simulink model "RLInvertedPendulumCtrl"  (R2017a)
settings: Solver=ode5  StartTime=0.0  StopTime=60  FixedStep=0.01  RelTol=1e-3
PreLoadFcn:
  | InvertedPendulumCtrlInit
values from neighbouring files (symbols this model uses):
  eta = 1.05    [InvertedPendulumSimCtrlInit.m]
  g = 9.81    [PendulumParameters.m]
  J = 0.0087878516209625    (= 0.00878785162096)    [PendulumParameters.m]
  K = lqr(A, B, Q, R)    [InvertedPendulumSimCtrlInit.m]
  kcw = 3    [InvertedPendulumSimCtrlInit.m]
  kem = 7    [InvertedPendulumSimCtrlInit.m]
  ksu = 1.3    [InvertedPendulumSimCtrlInit.m]
  kvw = 3    [InvertedPendulumSimCtrlInit.m]
  l = 0.2545253256150507    (= 0.254525325615)    [PendulumParameters.m]    (also in PlotPendulum.m = 1.8)
  mp = 0.096739999999999999    (= 0.09674)    [PendulumParameters.m]
  OffsetCart = 0    [PendulumParameters.m]
  OffsetPend = pi    (= 3.14159265359)    [PendulumParameters.m]
  ResCartEnc = 0.235 / 4096    (= 5.7373046875e-05)    [PendulumParameters.m]
  ResPendEnc = 2 * pi / 4096    (= 0.00153398078789)    [PendulumParameters.m]
  Td = 0.0    (= 0)    [InvertedPendulumSimCtrlInit.m]
  Ts = 0.01    [PendulumParameters.m]
  vmax = 5    [InvertedPendulumSimCtrlInit.m]
  x0 = [0; 0; pi + 0.01; 0]    [InvertedPendulumSimCtrlInit.m]
  xmax = 0.4    [InvertedPendulumSimCtrlInit.m]
undefined symbols (not defined in the file or in its folder): bias, bias0, bias2, bias4, M, sgn, weight0, weight2, weight4
undefined symbols (not defined in the file): angleSZ, Fs, RTDAC4PCIBaseAddress
libraries: simulink x1
settings Model: SimulationMode=external  ExtModeTrigDuration=12000  ExtModeTrigLevel=0.400000  Creator=jims  LastModifiedBy=Pendulum
settings DataIOCC: SaveFormat=Array  SaveOutput=off  SignalLogging=off  DSMLogging=off  SaveTime=off  SignalLoggingName=sigsOut
settings OptimizationCC: DefaultParameterBehavior=Inlined  InlineInvariantSignals=on  EfficientFloat2IntCast=on  SimCompilerOptimization=on
settings DebuggingCC: SaveWithParameterizedLinksMsg=none  IntegerOverflowMsg=none  UniqueDataStoreMsg=error  AssertControl=DisableAll  StrictBusMsg=ErrorOnBusTreatedAsVector  SFUnexpectedBacktrackingDiag=warning  SFNoUnconditionalDefaultTransitionDiag=warning  SFExecutionAtInitializationDiag=none  IntegerSaturationMsg=none
settings ModelReferenceCC: PropagateSignalLabelsOutOfModel=off
settings SFSimCC: SimParseCustomCode=off
settings RTWCC: SystemTargetFile=sldrt.tlc  TemplateMakefile=sldrt.tmf  Description=Simulink Desktop Real-Time  RTWCompilerOptimization=on
settings CodeAppCC: MaxIdLength=95
settings SimulinkDesktopRealTimeCC: TargetPreCompLibLocation=C:\Program Files\MATLAB\R2017a\toolbox\sldrt\lib\win64  TargetLangStandard=C89/C90 (ANSI)  SupportVariableSizeSignals=off
settings ConfigComp: CovMetricSettings=dw  CovHtmlReporting=on  CovSaveCumulativeToWorkspaceVar=on  CovSaveSingleToWorkspaceVar=on  CovExternalEMLEnable=off  CovSFcnEnable=off

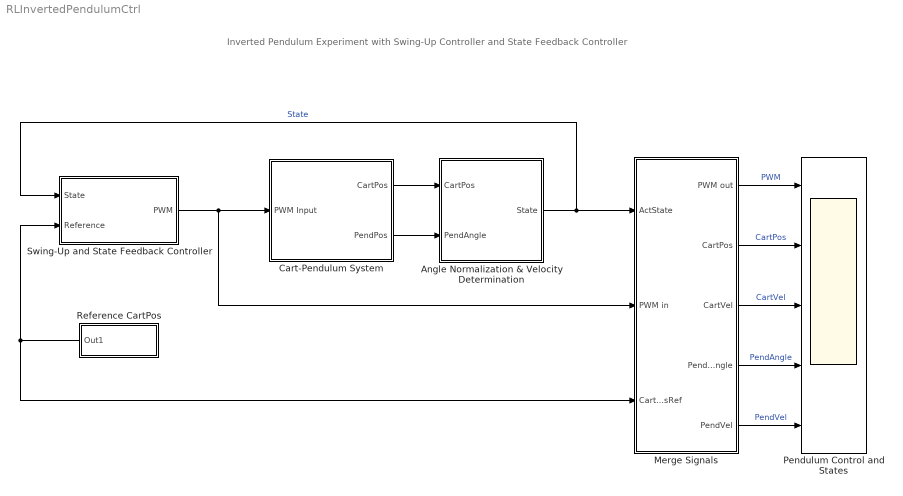
== system RLInvertedPendulumCtrl ==
  note: Inverted Pendulum Experiment with
      | Swing-Up Controller and State Feedback Controller
  Angle Normalization & Velocity Determination : Subsystem
  Cart-Pendulum System : Subsystem  mask(Cart-Pendulum System){BaseAddress=RTDAC4PCIBaseAddress(-1,-1)}
      mask prompts: BaseAddress "Base Address:"
      mask help: Interface to Cart-Pendulum System
      mask Display:
      | plot( [0.725 0.725], [1.15 0.375]); % pendulum arm
      | plot(0.725+0.05*sin([0:0.5:7]), 0.325+0.05*cos([0:0.5:7])); % pendulum load mass
      | plot([-0.2], [-0.2]);
      | plot([1.9], [1.7]);
      | plot([0.1 1.4], [1.09 1.09]); % upper rail
      | plot([0.1 1.4], [1.07 1.07]); % upper rail
      | plot([0.65 0.8], [1.1 1.1]); % cart bottom
      | plot([0.65 0.8], [1.2 1.2]); % cart top
      | plot([0.65 0.65], [1.2 1.1]); % cart left
      | plot([0.8 0.8], [1.1 1.2]); % cart right
      | port_label('input', 1, 'PWM');
      | port_label('output', 1, 'CartPos');
      | port_label('output', 2, 'PendAngle');
  Merge Signals : Subsystem
  Pendulum Control and States : Scope  NumInputPorts=5
  Reference CartPos : Subsystem  mask{Sine=off, Square=on, Sawtooth=off, Amplitude=0, Frequency=0.05}
      mask Display: disp('Generator')
  Swing-Up and State Feedback Controller : Subsystem
  wires:
  Merge Signals/2(CartPos) -> Pendulum Control and States/2  "CartPos"
  Merge Signals/3(CartVel) -> Pendulum Control and States/3  "CartVel"
  Merge Signals/4(PendAngle) -> Pendulum Control and States/4  "PendAngle"
  Merge Signals/5(PendVel) -> Pendulum Control and States/5  "PendVel"
  Reference CartPos/1(Out1) -> Swing-Up and State Feedback Controller/2(Reference), Merge Signals/3(CartPosRef)
  Swing-Up and State Feedback Controller/1(PWM) -> Cart-Pendulum System/1(PWM Input), Merge Signals/2(PWM in)
  Cart-Pendulum System/2(PendPos) -> Angle Normalization & Velocity Determination/2(PendAngle)
  Angle Normalization & Velocity Determination/1(State) -> Swing-Up and State Feedback Controller/1(State), Merge Signals/1(ActState)  "State"
  Merge Signals/1(PWM out) -> Pendulum Control and States/1  "PWM"
  Cart-Pendulum System/1(CartPos) -> Angle Normalization & Velocity Determination/1(CartPos)

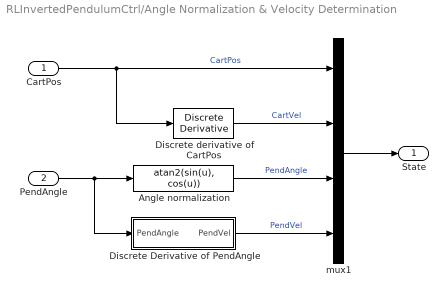
== system RLInvertedPendulumCtrl/Angle Normalization & Velocity Determination ==
  CartPos : Inport
  PendAngle : Inport  Port=2
  Angle normalization : Fcn  Expr=atan2(sin(u), cos(u))
  Discrete Derivative of PendAngle : Subsystem
  Discrete derivative of CartPos : simulink/Discrete/Discrete Derivative  gainval=1.0  ICPrevScaledInput=x0(1)/Ts  InputProcessing=Inherited  OutMin=[]  OutMax=[]  OutDataType=sfix(16)  OutScaling=2^-10  DoSatur=off
  mux1 : Mux
  State : Outport
  wires:
  Discrete Derivative of PendAngle/1(PendVel) -> mux1/4  "PendVel"
  Angle normalization/1 -> mux1/3  "PendAngle"
  Discrete derivative of CartPos/1 -> mux1/2  "CartVel"
  PendAngle/1 -> Discrete Derivative of PendAngle/1(PendAngle), Angle normalization/1
  mux1/1 -> State/1
  CartPos/1 -> mux1/1, Discrete derivative of CartPos/1  "CartPos"

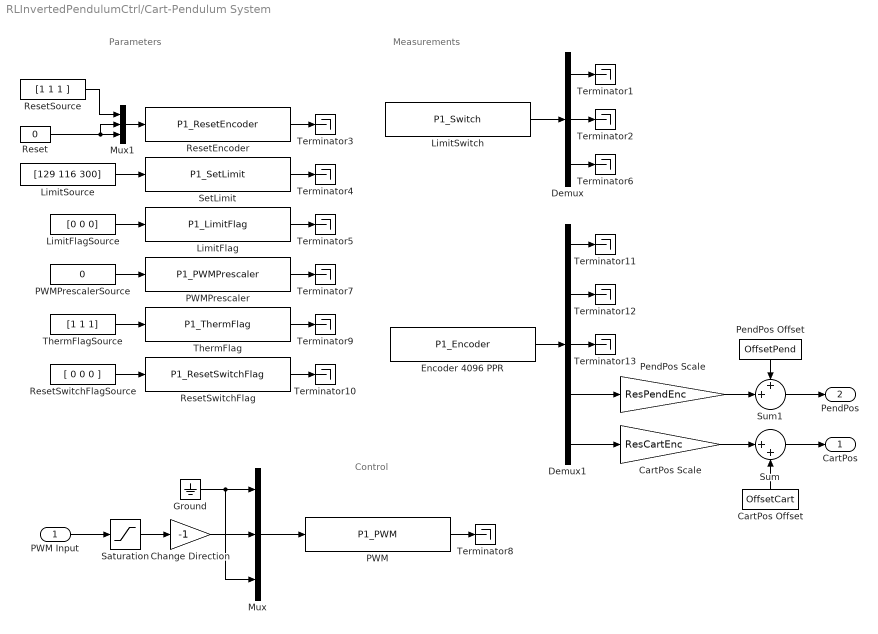
== system RLInvertedPendulumCtrl/Cart-Pendulum System ==
  note: Measurements
  note: Control
  note: Parameters
  PWM Input : Inport
  CartPos Offset : Constant  Value=OffsetCart
  CartPos Scale : Gain  Gain=ResCartEnc  OutDataTypeStr=Inherit: Same as input  ParamDataTypeStr=Inherit: Same as input
  Change Direction : Gain  Gain=-1  SaturateOnIntegerOverflow=on  OutDataTypeStr=Inherit: Same as input  ParamDataTypeStr=Inherit: Same as input
  Demux : Demux  Outputs=3
  Demux1 : Demux  Outputs=5
  Encoder 4096 PPR : S-Function  FunctionName=P1_Encoder  Parameters=BaseAddress, Ts  SFunctionDeploymentMode=off  EnableBusSupport=off
  Ground : Ground
  LimitFlag : S-Function  FunctionName=P1_LimitFlag  Parameters=BaseAddress, Ts  SFunctionDeploymentMode=off  EnableBusSupport=off
  LimitFlagSource : Constant  Value=[0 0 0]
  LimitSource : Constant  Value=[129 116 300]
  LimitSwitch : S-Function  FunctionName=P1_Switch  Parameters=BaseAddress, Ts  SFunctionDeploymentMode=off  EnableBusSupport=off
  Mux : Mux  Inputs=3
  Mux1 : Mux  Inputs=[3 1 1]
  PWM : S-Function  FunctionName=P1_PWM  Parameters=BaseAddress, Ts  SFunctionDeploymentMode=off  EnableBusSupport=off
  PWMPrescaler : S-Function  FunctionName=P1_PWMPrescaler  Parameters=BaseAddress, Ts  SFunctionDeploymentMode=off  EnableBusSupport=off
  PWMPrescalerSource : Constant  Value=0
  PendPos Offset : Constant  Value=OffsetPend
  PendPos Scale : Gain  Gain=ResPendEnc  OutDataTypeStr=Inherit: Same as input  ParamDataTypeStr=Inherit: Same as input
  Reset : Constant  Value=0
  ResetEncoder : S-Function  FunctionName=P1_ResetEncoder  Parameters=BaseAddress, Ts  SFunctionDeploymentMode=off  EnableBusSupport=off
  ResetSource : Constant  Value=[1 1 1 ]
  "ResetSwitchFlag " : S-Function  FunctionName=P1_ResetSwitchFlag  Parameters=BaseAddress, Ts  SFunctionDeploymentMode=off  EnableBusSupport=off
  ResetSwitchFlagSource : Constant  Value=[ 0 0 0 ]
  Saturation : Saturate
  SetLimit : S-Function  FunctionName=P1_SetLimit  Parameters=BaseAddress, Ts  SFunctionDeploymentMode=off  EnableBusSupport=off
  Sum : Sum  Inputs=|++  SaturateOnIntegerOverflow=on  InputSameDT=on  OutDataTypeStr=Inherit: Same as first input
  Sum1 : Sum  Inputs=++|  SaturateOnIntegerOverflow=on  InputSameDT=on  OutDataTypeStr=Inherit: Same as first input
  Terminator{1..13} (13 alike) : Terminator
  "ThermFlag " : S-Function  FunctionName=P1_ThermFlag  Parameters=BaseAddress, Ts  SFunctionDeploymentMode=off  EnableBusSupport=off
  ThermFlagSource : Constant  Value=[1 1 1]
  CartPos : Outport
  PendPos : Outport  Port=2
  wires:
  Demux1/1 -> Terminator11/1
  Demux1/2 -> Terminator12/1
  Demux1/3 -> Terminator13/1
  Demux1/4 -> PendPos Scale/1
  Demux1/5 -> CartPos Scale/1
  Demux/3 -> Terminator6/1
  Demux/2 -> Terminator2/1
  Demux/1 -> Terminator1/1
  LimitSwitch/1 -> Demux/1
  Ground/1 -> Mux/1, Mux/3
  ResetSwitchFlagSource/1 -> "ResetSwitchFlag "/1
  ThermFlagSource/1 -> "ThermFlag "/1
  PWMPrescalerSource/1 -> PWMPrescaler/1
  LimitFlagSource/1 -> LimitFlag/1
  LimitSource/1 -> SetLimit/1
  "ResetSwitchFlag "/1 -> Terminator10/1
  "ThermFlag "/1 -> Terminator9/1
  PWMPrescaler/1 -> Terminator7/1
  LimitFlag/1 -> Terminator5/1
  SetLimit/1 -> Terminator4/1
  ResetEncoder/1 -> Terminator3/1
  PWM/1 -> Terminator8/1
  Mux/1 -> PWM/1
  Encoder 4096 PPR/1 -> Demux1/1
  Mux1/1 -> ResetEncoder/1
  ResetSource/1 -> Mux1/1
  Change Direction/1 -> Mux/2
  PWM Input/1 -> Saturation/1
  PendPos Scale/1 -> Sum1/2
  PendPos Offset/1 -> Sum1/1
  Reset/1 -> Mux1/2, Mux1/3
  Saturation/1 -> Change Direction/1
  CartPos Offset/1 -> Sum/2
  CartPos Scale/1 -> Sum/1
  Sum/1 -> CartPos/1
  Sum1/1 -> PendPos/1

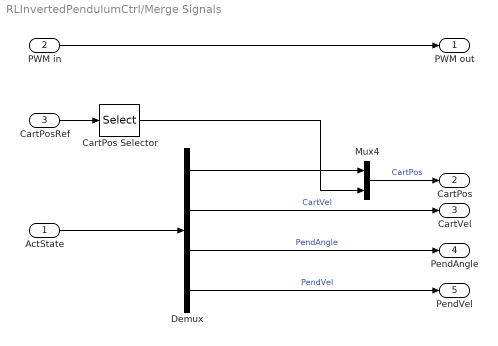
== system RLInvertedPendulumCtrl/Merge Signals ==
  ActState : Inport
  PWM in : Inport  Port=2
  CartPosRef : Inport  Port=3
  CartPos Selector : Selector  InputPortWidth=4  IndexOptions=Index vector (dialog)  Indices=[1]  OutputSizes=1
  Demux : Demux
  Mux4 : Mux  Inputs=2
  PWM out : Outport
  CartPos : Outport  Port=2
  CartVel : Outport  Port=3
  PendAngle : Outport  Port=4
  PendVel : Outport  Port=5
  wires:
  Mux4/1 -> CartPos/1  "CartPos"
  Demux/2 -> CartVel/1  "CartVel"
  Demux/3 -> PendAngle/1  "PendAngle"
  Demux/4 -> PendVel/1  "PendVel"
  Demux/1 -> Mux4/1
  CartPosRef/1 -> CartPos Selector/1
  ActState/1 -> Demux/1
  CartPos Selector/1 -> Mux4/2
  PWM in/1 -> PWM out/1

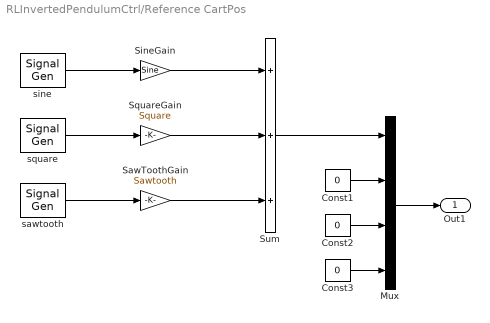
== system RLInvertedPendulumCtrl/Reference CartPos ==
  Const1 : Constant  Value=0
  Const2 : Constant  Value=0
  Const3 : Constant  Value=0
  Mux : Mux
  SawToothGain : Gain  Gain=Sawtooth  SaturateOnIntegerOverflow=on  OutDataTypeStr=Inherit: Same as input  ParamDataTypeStr=Inherit: Same as input
  SineGain : Gain  Gain=Sine  SaturateOnIntegerOverflow=on  OutDataTypeStr=Inherit: Same as input  ParamDataTypeStr=Inherit: Same as input
  SquareGain : Gain  Gain=Square  SaturateOnIntegerOverflow=on  OutDataTypeStr=Inherit: Same as input  ParamDataTypeStr=Inherit: Same as input
  Sum : Sum  Inputs=+++  SaturateOnIntegerOverflow=on  InputSameDT=on  OutDataTypeStr=Inherit: Same as first input
  sawtooth : SignalGenerator  WaveForm=sawtooth  Amplitude=Amplitude  Frequency=Frequency
  sine : SignalGenerator  Amplitude=Amplitude  Frequency=Frequency
  square : SignalGenerator  WaveForm=square  Amplitude=Amplitude  Frequency=Frequency
  Out1 : Outport
  wires:
  SawToothGain/1 -> Sum/3
  SquareGain/1 -> Sum/2
  SineGain/1 -> Sum/1
  sawtooth/1 -> SawToothGain/1
  square/1 -> SquareGain/1
  sine/1 -> SineGain/1
  Const2/1 -> Mux/3
  Const3/1 -> Mux/4
  Mux/1 -> Out1/1
  Const1/1 -> Mux/2
  Sum/1 -> Mux/1

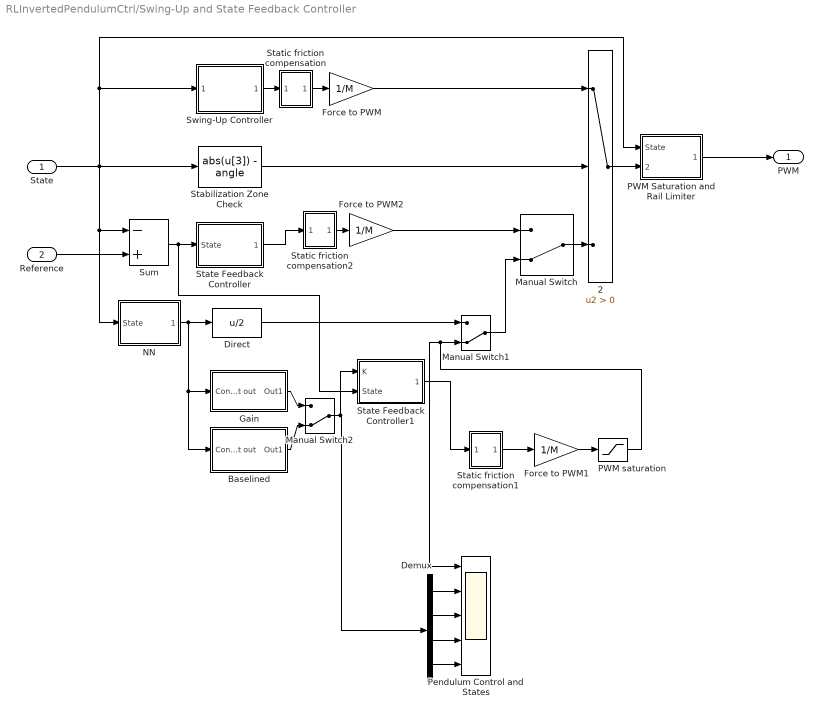
== system RLInvertedPendulumCtrl/Swing-Up and State Feedback Controller ==
  State : Inport
  Reference : Inport  Port=2
  2 : Switch  Criteria=u2 > Threshold  SaturateOnIntegerOverflow=on  InputSameDT=on
  Baselined : Subsystem
  Demux : Demux
  Direct : Fcn  Expr=u/2
  Force to PWM : Gain  Gain=1/M  SaturateOnIntegerOverflow=on  OutDataTypeStr=Inherit: Same as input  ParamDataTypeStr=Inherit: Same as input
  Force to PWM1 : Gain  Gain=1/M  SaturateOnIntegerOverflow=on  OutDataTypeStr=Inherit: Same as input  ParamDataTypeStr=Inherit: Same as input
  Force to PWM2 : Gain  Gain=1/M  SaturateOnIntegerOverflow=on  OutDataTypeStr=Inherit: Same as input  ParamDataTypeStr=Inherit: Same as input
  Gain : Subsystem
  Manual Switch : ManualSwitch  CurrentSetting=0
  Manual Switch1 : ManualSwitch  CurrentSetting=0
  Manual Switch2 : ManualSwitch  CurrentSetting=0
  NN : Subsystem
  PWM saturation : Saturate
  PWM Saturation and Rail Limiter : Subsystem  mask(State feedback controller){}
      mask Display: plot(0,0,100,100,[10,90,90,10],[52,52,50,50],[30,30],[52,60],[70,68,68,70,70],[60,60,52,52,60],[30,32,32,30],[52,52,60,60])
  Pendulum Control and States : Scope  NumInputPorts=5
  Stabilization Zone Check : Fcn  Expr=abs(u[3]) - angle  mask(Stabilization zone check){angle=angleSZ}
      mask prompts: angle "stabilization zone angle [rad]"
      mask help: Check if pendulum is insidde stabilization zone: abs(theta) <= angle
      mask Display: plot(0,0,100,100,[40,60,80,83,80,60,40,20,17,20,40],[89,89,80,70,60,51,51,60,69,80,90],[83,50,17],[70,8,68])
  State Feedback Controller : Subsystem  mask(State feedback controller){}
      mask Display: plot(0,0,100,100,[40,30,20],[87,85,80],[46,54,54,46,46],[90,90,80,80,90],[46,45,45,46,54,55,55,54,46],[78,80,90,91,91,90,80,78,78],[51,51,49,49],[78,10,10,78],[90,80,70,60],[70,80,85,88],[20,10],[80,70],[20,20,15],[73,80,80],[85,80,80],[80,80,74])
  State Feedback Controller1 : Subsystem  mask(State feedback controller){}
      mask Display: plot(0,0,100,100,[40,30,20],[87,85,80],[46,54,54,46,46],[90,90,80,80,90],[46,45,45,46,54,55,55,54,46],[78,80,90,91,91,90,80,78,78],[51,51,49,49],[78,10,10,78],[90,80,70,60],[70,80,85,88],[20,10],[80,70],[20,20,15],[73,80,80],[85,80,80],[80,80,74])
  Static friction compensation : Subsystem  mask(Static Friction){f=Fs}
      mask prompts: f "Static friction (f)"
      mask help:
      | A discontinuity offset at zero models static friction
      | y = u + sgn(u)*f
      mask Display: plot([-1 0 0 1],[-f-1, -f, f, 1+f],[-1 1],[0 0],[0 0],[-f,f])
  Static friction compensation1 : Subsystem  mask(Static Friction){f=Fs}
      mask prompts: f "Static friction (f)"
      mask help:
      | A discontinuity offset at zero models static friction
      | y = u + sgn(u)*f
      mask Display: plot([-1 0 0 1],[-f-1, -f, f, 1+f],[-1 1],[0 0],[0 0],[-f,f])
  Static friction compensation2 : Subsystem  mask(Static Friction){f=Fs}
      mask prompts: f "Static friction (f)"
      mask help:
      | A discontinuity offset at zero models static friction
      | y = u + sgn(u)*f
      mask Display: plot([-1 0 0 1],[-f-1, -f, f, 1+f],[-1 1],[0 0],[0 0],[-f,f])
  Sum : Sum  Inputs=-+  SaturateOnIntegerOverflow=on
  Swing-Up Controller : Subsystem  mask(Swing-up Controller){}
      mask Display: plot(0,0,100,100,[20,20],[12,87],[93,90,90,93,7],[50,46,54,50,50],[20,22,18,20],[87,80,80,88],[80,80,75,75,71,71,65,65,60,60,49,49,40,40,20],[50,40,40,60,60,50,50,80,80,20,21,80,80,21,20])
  PWM : Outport
  wires:
  Stabilization Zone Check/1 -> 2/2
  Sum/1 -> State Feedback Controller1/2(State), State Feedback Controller/1(State)
  State/1 -> NN/1(State), Sum/1, Swing-Up Controller/1(States), PWM Saturation and Rail Limiter/1(State), Stabilization Zone Check/1
  Reference/1 -> Sum/2
  PWM Saturation and Rail Limiter/1(Control input out) -> PWM/1
  Force to PWM/1 -> 2/1
  Swing-Up Controller/1(Control) -> Static friction compensation/1(In1)
  Static friction compensation/1(Out1) -> Force to PWM/1
  2/1 -> PWM Saturation and Rail Limiter/2(Control input in)
  State Feedback Controller/1(Control input) -> Static friction compensation2/1(In1)
  Manual Switch/1 -> 2/3
  Static friction compensation1/1(Out1) -> Force to PWM1/1
  Direct/1 -> Manual Switch1/1
  Manual Switch1/1 -> Manual Switch/2
  State Feedback Controller1/1(Control input) -> Static friction compensation1/1(In1)
  Static friction compensation2/1(Out1) -> Force to PWM2/1
  Force to PWM2/1 -> Manual Switch/1
  Demux/1 -> Pendulum Control and States/2
  Demux/2 -> Pendulum Control and States/3
  Demux/3 -> Pendulum Control and States/4
  Demux/4 -> Pendulum Control and States/5
  Force to PWM1/1 -> PWM saturation/1
  PWM saturation/1 -> Manual Switch1/2, Pendulum Control and States/1
  Gain/1(Out1) -> Manual Switch2/1
  Baselined/1(Out1) -> Manual Switch2/2
  Manual Switch2/1 -> State Feedback Controller1/1(K), Demux/1
  NN/1(Control input out) -> Baselined/1(Control input out), Gain/1(Control input out), Direct/1

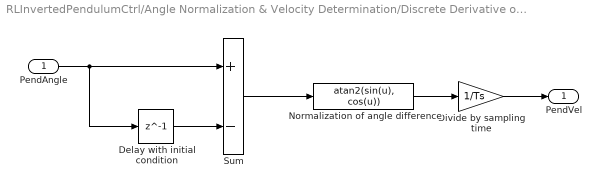
== system RLInvertedPendulumCtrl/Angle Normalization & Velocity Determination/Discrete Derivative of PendAngle ==
  PendAngle : Inport
  Delay with initial condition : Delay  DelayLength=1  InitialCondition=x0(3)
  Divide by sampling time : Gain  Gain=1/Ts
  Normalization of angle difference : Fcn  Expr=atan2(sin(u), cos(u))
  Sum : Sum  Inputs=+-
  PendVel : Outport
  wires:
  Sum/1 -> Normalization of angle difference/1
  Normalization of angle difference/1 -> Divide by sampling time/1
  Divide by sampling time/1 -> PendVel/1
  PendAngle/1 -> Delay with initial condition/1, Sum/1
  Delay with initial condition/1 -> Sum/2

== system RLInvertedPendulumCtrl/Swing-Up and State Feedback Controller/Baselined ==
  Control input out : Inport
  Add : Sum
  Constant : Constant  Value=K
  Product : Product
  Out1 : Outport
  wires:
  Add/1 -> Out1/1
  Constant/1 -> Product/1, Add/1
  Product/1 -> Add/2
  Control input out/1 -> Product/2

== system RLInvertedPendulumCtrl/Swing-Up and State Feedback Controller/Gain ==
  Control input out : Inport
  Constant : Constant
  Constant1 : Constant  Value=50
  Product1 : Product
  Subtract : Sum  Inputs=+-
  Out1 : Outport
  wires:
  Constant/1 -> Subtract/2
  Subtract/1 -> Product1/1
  Constant1/1 -> Product1/2
  Control input out/1 -> Subtract/1
  Product1/1 -> Out1/1

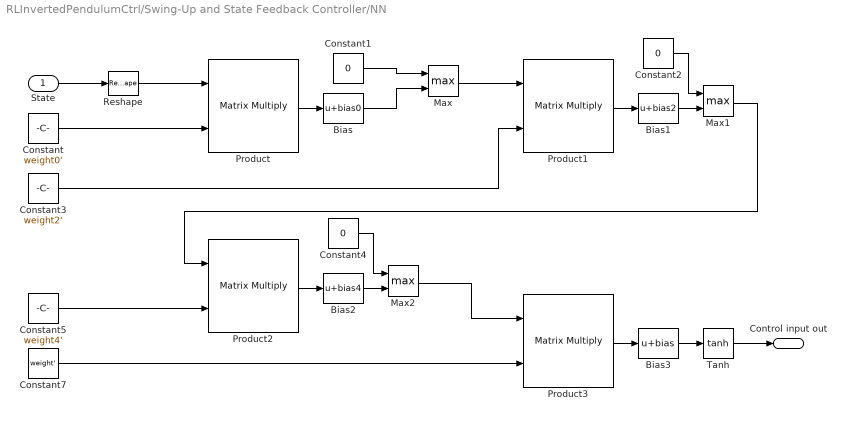
== system RLInvertedPendulumCtrl/Swing-Up and State Feedback Controller/NN ==
  State : Inport
  Bias : Bias  Bias=bias0
  Bias1 : Bias  Bias=bias2
  Bias2 : Bias  Bias=bias4
  Bias3 : Bias  Bias=bias
  Constant : Constant  Value=weight0'
  Constant1 : Constant  Value=0
  Constant2 : Constant  Value=0
  Constant3 : Constant  Value=weight2'
  Constant4 : Constant  Value=0
  Constant5 : Constant  Value=weight4'
  Constant7 : Constant  Value=weight'
  Max : MinMax  Function=max  Inputs=2
  Max1 : MinMax  Function=max  Inputs=2
  Max2 : MinMax  Function=max  Inputs=2
  Product{,1..3} (4 alike) : Product  Multiplication=Matrix(*)
  Reshape : Reshape  OutputDimensionality=Row vector (2-D)
  Tanh : Trigonometry  Operator=tanh
  Control input out : Outport
  wires:
  Constant7/1 -> Product3/2
  Constant3/1 -> Product1/2
  Max1/1 -> Product2/1
  Bias1/1 -> Max1/2
  Max2/1 -> Product3/1
  Constant1/1 -> Max/1
  Bias3/1 -> Tanh/1
  Product1/1 -> Bias1/1
  Max/1 -> Product1/1
  Bias/1 -> Max/2
  Constant4/1 -> Max2/1
  Constant2/1 -> Max1/1
  Tanh/1 -> Control input out/1
  Product3/1 -> Bias3/1
  Constant/1 -> Product/2
  Bias2/1 -> Max2/2
  Constant5/1 -> Product2/2
  Product/1 -> Bias/1
  State/1 -> Reshape/1
  Product2/1 -> Bias2/1
  Reshape/1 -> Product/1

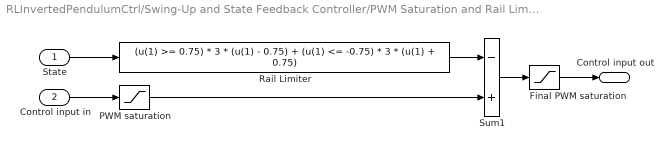
== system RLInvertedPendulumCtrl/Swing-Up and State Feedback Controller/PWM Saturation and Rail Limiter ==
  State : Inport
  Control input in : Inport  Port=2
  Final PWM saturation : Saturate
  PWM saturation : Saturate
  Rail Limiter : Fcn  Expr=(u(1) >= 0.75) * 3 * (u(1) - 0.75) + (u(1) <= -0.75) * 3 * (u(1) + 0.75)
  Sum1 : Sum  Inputs=-+  SaturateOnIntegerOverflow=on  InputSameDT=on  OutDataTypeStr=Inherit: Same as first input
  Control input out : Outport
  wires:
  State/1 -> Rail Limiter/1
  Rail Limiter/1 -> Sum1/1
  Control input in/1 -> PWM saturation/1
  Sum1/1 -> Final PWM saturation/1
  PWM saturation/1 -> Sum1/2
  Final PWM saturation/1 -> Control input out/1

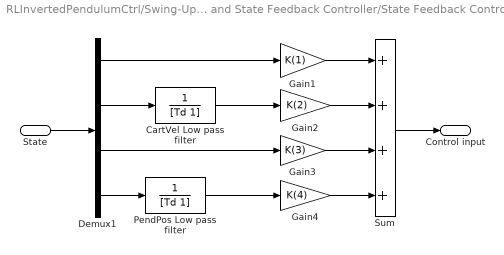
== system RLInvertedPendulumCtrl/Swing-Up and State Feedback Controller/State Feedback Controller ==
  State : Inport
  CartVel Low pass filter : TransferFcn  Denominator=[Td 1]
  Demux1 : Demux
  Gain1 : Gain  Gain=K(1)  SaturateOnIntegerOverflow=on  OutDataTypeStr=Inherit: Same as input  ParamDataTypeStr=Inherit: Same as input
  Gain2 : Gain  Gain=K(2)  SaturateOnIntegerOverflow=on  OutDataTypeStr=Inherit: Same as input  ParamDataTypeStr=Inherit: Same as input
  Gain3 : Gain  Gain=K(3)  SaturateOnIntegerOverflow=on  OutDataTypeStr=Inherit: Same as input  ParamDataTypeStr=Inherit: Same as input
  Gain4 : Gain  Gain=K(4)  SaturateOnIntegerOverflow=on  OutDataTypeStr=Inherit: Same as input  ParamDataTypeStr=Inherit: Same as input
  PendPos Low pass filter : TransferFcn  Denominator=[Td 1]
  Sum : Sum  Inputs=++++  SaturateOnIntegerOverflow=on  InputSameDT=on  OutDataTypeStr=Inherit: Same as first input
  Control input : Outport
  wires:
  Demux1/1 -> Gain1/1
  Gain1/1 -> Sum/1
  Gain2/1 -> Sum/2
  Demux1/2 -> CartVel Low pass filter/1
  Gain3/1 -> Sum/3
  Demux1/3 -> Gain3/1
  Gain4/1 -> Sum/4
  Demux1/4 -> PendPos Low pass filter/1
  Sum/1 -> Control input/1
  State/1 -> Demux1/1
  PendPos Low pass filter/1 -> Gain4/1
  CartVel Low pass filter/1 -> Gain2/1

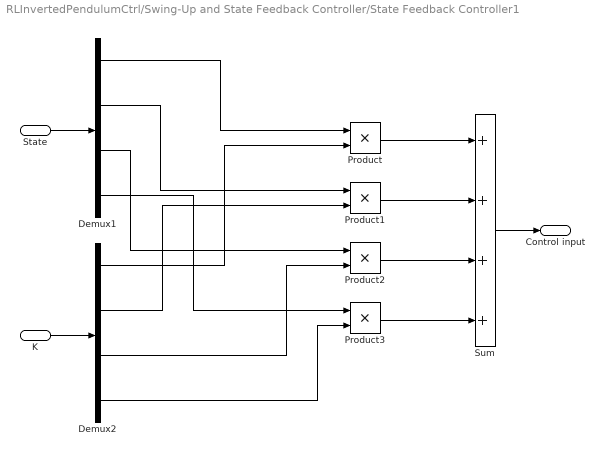
== system RLInvertedPendulumCtrl/Swing-Up and State Feedback Controller/State Feedback Controller1 ==
  K : Inport
  State : Inport  Port=2
  Demux1 : Demux
  Demux2 : Demux
  Product{,1..3} (4 alike) : Product
  Sum : Sum  Inputs=++++  SaturateOnIntegerOverflow=on  InputSameDT=on  OutDataTypeStr=Inherit: Same as first input
  Control input : Outport
  wires:
  Sum/1 -> Control input/1
  State/1 -> Demux1/1
  K/1 -> Demux2/1
  Demux1/1 -> Product/1
  Demux2/1 -> Product/2
  Demux1/2 -> Product1/1
  Demux2/2 -> Product1/2
  Demux1/3 -> Product2/1
  Demux2/3 -> Product2/2
  Demux1/4 -> Product3/1
  Demux2/4 -> Product3/2
  Product/1 -> Sum/1
  Product1/1 -> Sum/2
  Product2/1 -> Sum/3
  Product3/1 -> Sum/4

== system RLInvertedPendulumCtrl/Swing-Up and State Feedback Controller/Static friction compensation ==
  In1 : Inport
  Gain1 : Gain  Gain=f  SaturateOnIntegerOverflow=on  OutDataTypeStr=Inherit: Same as input  ParamDataTypeStr=Inherit: Same as input
  Sign : Signum
  Sum : Sum  Inputs=|++  SaturateOnIntegerOverflow=on  InputSameDT=on  OutDataTypeStr=Inherit: Same as first input
  Out1 : Outport
  wires:
  Sign/1 -> Gain1/1
  In1/1 -> Sign/1, Sum/2
  Gain1/1 -> Sum/1
  Sum/1 -> Out1/1

== system RLInvertedPendulumCtrl/Swing-Up and State Feedback Controller/Static friction compensation1 ==
  In1 : Inport
  Gain1 : Gain  Gain=f  SaturateOnIntegerOverflow=on  OutDataTypeStr=Inherit: Same as input  ParamDataTypeStr=Inherit: Same as input
  Sign : Signum
  Sum : Sum  Inputs=|++  SaturateOnIntegerOverflow=on  InputSameDT=on  OutDataTypeStr=Inherit: Same as first input
  Out1 : Outport
  wires:
  Sign/1 -> Gain1/1
  In1/1 -> Sign/1, Sum/2
  Gain1/1 -> Sum/1
  Sum/1 -> Out1/1

== system RLInvertedPendulumCtrl/Swing-Up and State Feedback Controller/Static friction compensation2 ==
  In1 : Inport
  Gain1 : Gain  Gain=f  SaturateOnIntegerOverflow=on  OutDataTypeStr=Inherit: Same as input  ParamDataTypeStr=Inherit: Same as input
  Sign : Signum
  Sum : Sum  Inputs=|++  SaturateOnIntegerOverflow=on  InputSameDT=on  OutDataTypeStr=Inherit: Same as first input
  Out1 : Outport
  wires:
  Sign/1 -> Gain1/1
  In1/1 -> Sign/1, Sum/2
  Gain1/1 -> Sum/1
  Sum/1 -> Out1/1

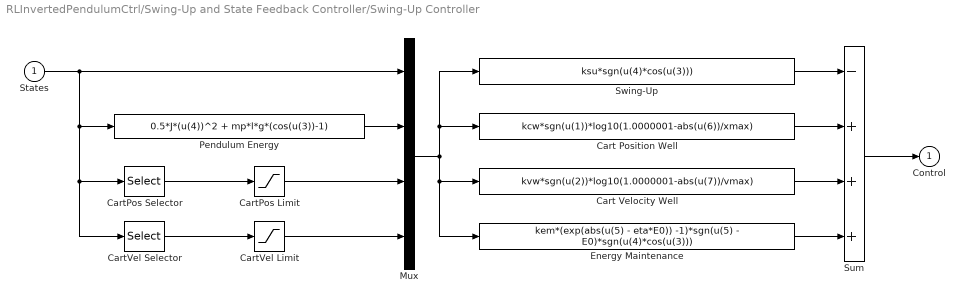
== system RLInvertedPendulumCtrl/Swing-Up and State Feedback Controller/Swing-Up Controller ==
  States : Inport
  Cart Position Well : Fcn  Expr=kcw*sgn(u(1))*log10(1.0000001-abs(u(6))/xmax)
  Cart Velocity Well : Fcn  Expr=kvw*sgn(u(2))*log10(1.0000001-abs(u(7))/vmax)
  CartPos Limit : Saturate  UpperLimit=xmax  LowerLimit=-xmax
  CartPos Selector : Selector  InputPortWidth=4  IndexOptions=Index vector (dialog)  Indices=[1]  OutputSizes=1
  CartVel Limit : Saturate  UpperLimit=vmax  LowerLimit=-vmax
  CartVel Selector : Selector  InputPortWidth=4  IndexOptions=Index vector (dialog)  Indices=[2]  OutputSizes=1
  Energy Maintenance : Fcn  Expr=kem*(exp(abs(u(5) - eta*E0)) -1)*sgn(u(5) - E0)*sgn(u(4)*cos(u(3)))
  Mux : Mux
  Pendulum Energy : Fcn  Expr=0.5*J*(u(4))^2 + mp*l*g*(cos(u(3))-1)
  Sum : Sum  Inputs=-+++  SaturateOnIntegerOverflow=on
  Swing-Up : Fcn  Expr=ksu*sgn(u(4)*cos(u(3)))
  Control : Outport
  wires:
  States/1 -> Mux/1, Pendulum Energy/1, CartPos Selector/1, CartVel Selector/1
  Pendulum Energy/1 -> Mux/2
  CartPos Selector/1 -> CartPos Limit/1
  CartPos Limit/1 -> Mux/3
  CartVel Selector/1 -> CartVel Limit/1
  CartVel Limit/1 -> Mux/4
  Mux/1 -> Swing-Up/1, Cart Position Well/1, Cart Velocity Well/1, Energy Maintenance/1
  Sum/1 -> Control/1
  Swing-Up/1 -> Sum/1
  Cart Position Well/1 -> Sum/2
  Cart Velocity Well/1 -> Sum/3
  Energy Maintenance/1 -> Sum/4
